simulink library "powerlib2"  (Simulink 6.0)
settings: Solver=ode45  SolverMode=SingleTasking  StartTime=0.0  StopTime=10.0  RelTol=1e-3
undefined symbols (not defined in the file or in its folder): com, ctrl1, Da, DiscIntNeverNeededParam, dtha, etat, FA, gcbh, Ha, Ka, Lm, Ls, powericonV2, q0, Rm, Rs, sel, st_a, st_b, st_c, sta, stb, stc, T1, T2, T3, T4
libraries: powerlib2 x55, simulink_extras x5, powerlib_extras x4, powerlib_modelsV2 x4, simulink x1
(part 6 of 6)

== system powerlib2/Machines/STG/4 mass shaft/2 masses/Mass2 ==
  Ts_k+1 : Inport  Port=1  LatchInput=off
  Tt_k : Inport  Port=2  LatchInput=off
  deltat_k-1 : Inport  Port=3  LatchInput=off
  Gain10 : Gain  Gain=D  SaturateOnIntegerOverflow=on
  Gain11 : Gain  Gain=K  SaturateOnIntegerOverflow=on
  Gain9 : Gain  Gain=1/(2*H)  SaturateOnIntegerOverflow=on
  Integrator6 : Integrator
  Integrator7 : Integrator  InitialCondition=dth0
  Sum11 : Sum  Orientation=left  Inputs=|+-  SaturateOnIntegerOverflow=on  InputSameDT=on
  Sum9 : Sum  Inputs=+|+|-|-  SaturateOnIntegerOverflow=on  InputSameDT=on
  pu2radpersec : Gain  Gain=120*pi  SaturateOnIntegerOverflow=on
  deltat_k : Outport  InitialOutput=0
  Ts_k : Outport  Port=2  InitialOutput=0
  dw : Outport  Port=3  InitialOutput=0
  wires:
  deltat_k-1/1 -> Sum11/2
  Sum11/1 -> Gain11/1
  Integrator7/1 -> deltat_k/1, Sum11/1
  pu2radpersec/1 -> Integrator7/1
  Integrator6/1 -> pu2radpersec/1, Gain10/1, dw/1
  Tt_k/1 -> Sum9/2
  Sum9/1 -> Gain9/1
  Gain10/1 -> Sum9/4
  Gain11/1 -> Ts_k/1, Sum9/3
  Ts_k+1/1 -> Sum9/1
  Gain9/1 -> Integrator6/1

== system powerlib2/Machines/STG/4 mass shaft/2 masses/Mass3 ==
  Ts_k+1 : Inport  Port=1  LatchInput=off
  Tt_k : Inport  Port=2  LatchInput=off
  deltat_k-1 : Inport  Port=3  LatchInput=off
  Gain10 : Gain  Gain=D  SaturateOnIntegerOverflow=on
  Gain11 : Gain  Gain=K  SaturateOnIntegerOverflow=on
  Gain9 : Gain  Gain=1/(2*H)  SaturateOnIntegerOverflow=on
  Integrator6 : Integrator
  Integrator7 : Integrator  InitialCondition=dth0
  Sum11 : Sum  Orientation=left  Inputs=|+-  SaturateOnIntegerOverflow=on  InputSameDT=on
  Sum9 : Sum  Inputs=+|+|-|-  SaturateOnIntegerOverflow=on  InputSameDT=on
  pu2radpersec : Gain  Gain=120*pi  SaturateOnIntegerOverflow=on
  deltat_k : Outport  InitialOutput=0
  Ts_k : Outport  Port=2  InitialOutput=0
  dw : Outport  Port=3  InitialOutput=0
  wires:
  Ts_k+1/1 -> Sum9/1
  Gain11/1 -> Sum9/3, Ts_k/1
  Gain10/1 -> Sum9/4
  Sum9/1 -> Gain9/1
  Gain9/1 -> Integrator6/1
  Tt_k/1 -> Sum9/2
  Integrator6/1 -> pu2radpersec/1, Gain10/1, dw/1
  pu2radpersec/1 -> Integrator7/1
  Integrator7/1 -> Sum11/1, deltat_k/1
  Sum11/1 -> Gain11/1
  deltat_k-1/1 -> Sum11/2

== system powerlib2/Machines/STG/4 mass shaft/3 masses/Mass2 ==
  Ts_k+1 : Inport  Port=1  LatchInput=off
  Tt_k : Inport  Port=2  LatchInput=off
  deltat_k-1 : Inport  Port=3  LatchInput=off
  Gain10 : Gain  Gain=D  SaturateOnIntegerOverflow=on
  Gain11 : Gain  Gain=K  SaturateOnIntegerOverflow=on
  Gain9 : Gain  Gain=1/(2*H)  SaturateOnIntegerOverflow=on
  Integrator6 : Integrator
  Integrator7 : Integrator  InitialCondition=dth0
  Sum11 : Sum  Orientation=left  Inputs=|+-  SaturateOnIntegerOverflow=on  InputSameDT=on
  Sum9 : Sum  Inputs=+|+|-|-  SaturateOnIntegerOverflow=on  InputSameDT=on
  pu2radpersec : Gain  Gain=120*pi  SaturateOnIntegerOverflow=on
  deltat_k : Outport  InitialOutput=0
  Ts_k : Outport  Port=2  InitialOutput=0
  dw : Outport  Port=3  InitialOutput=0
  wires:
  deltat_k-1/1 -> Sum11/2
  Sum11/1 -> Gain11/1
  Integrator7/1 -> deltat_k/1, Sum11/1
  pu2radpersec/1 -> Integrator7/1
  Integrator6/1 -> pu2radpersec/1, Gain10/1, dw/1
  Tt_k/1 -> Sum9/2
  Sum9/1 -> Gain9/1
  Gain10/1 -> Sum9/4
  Gain11/1 -> Ts_k/1, Sum9/3
  Ts_k+1/1 -> Sum9/1
  Gain9/1 -> Integrator6/1

== system powerlib2/Machines/STG/4 mass shaft/3 masses/Mass3 ==
  Ts_k+1 : Inport  Port=1  LatchInput=off
  Tt_k : Inport  Port=2  LatchInput=off
  deltat_k-1 : Inport  Port=3  LatchInput=off
  Gain10 : Gain  Gain=D  SaturateOnIntegerOverflow=on
  Gain11 : Gain  Gain=K  SaturateOnIntegerOverflow=on
  Gain9 : Gain  Gain=1/(2*H)  SaturateOnIntegerOverflow=on
  Integrator6 : Integrator
  Integrator7 : Integrator  InitialCondition=dth0
  Sum11 : Sum  Orientation=left  Inputs=|+-  SaturateOnIntegerOverflow=on  InputSameDT=on
  Sum9 : Sum  Inputs=+|+|-|-  SaturateOnIntegerOverflow=on  InputSameDT=on
  pu2radpersec : Gain  Gain=120*pi  SaturateOnIntegerOverflow=on
  deltat_k : Outport  InitialOutput=0
  Ts_k : Outport  Port=2  InitialOutput=0
  dw : Outport  Port=3  InitialOutput=0
  wires:
  Ts_k+1/1 -> Sum9/1
  Gain11/1 -> Sum9/3, Ts_k/1
  Gain10/1 -> Sum9/4
  Sum9/1 -> Gain9/1
  Gain9/1 -> Integrator6/1
  Tt_k/1 -> Sum9/2
  Integrator6/1 -> pu2radpersec/1, Gain10/1, dw/1
  pu2radpersec/1 -> Integrator7/1
  Integrator7/1 -> Sum11/1, deltat_k/1
  Sum11/1 -> Gain11/1
  deltat_k-1/1 -> Sum11/2

== system powerlib2/Machines/STG/4 mass shaft/3 masses/Mass4 ==
  Ts_k+1 : Inport  Port=1  LatchInput=off
  Tt_k : Inport  Port=2  LatchInput=off
  deltat_k-1 : Inport  Port=3  LatchInput=off
  Gain10 : Gain  Gain=D  SaturateOnIntegerOverflow=on
  Gain11 : Gain  Gain=K  SaturateOnIntegerOverflow=on
  Gain9 : Gain  Gain=1/(2*H)  SaturateOnIntegerOverflow=on
  Integrator6 : Integrator
  Integrator7 : Integrator  InitialCondition=dth0
  Sum11 : Sum  Orientation=left  Inputs=|+-  SaturateOnIntegerOverflow=on  InputSameDT=on
  Sum9 : Sum  Inputs=+|+|-|-  SaturateOnIntegerOverflow=on  InputSameDT=on
  pu2radpersec : Gain  Gain=120*pi  SaturateOnIntegerOverflow=on
  deltat_k : Outport  InitialOutput=0
  Ts_k : Outport  Port=2  InitialOutput=0
  dw : Outport  Port=3  InitialOutput=0
  wires:
  deltat_k-1/1 -> Sum11/2
  Sum11/1 -> Gain11/1
  Integrator7/1 -> deltat_k/1, Sum11/1
  pu2radpersec/1 -> Integrator7/1
  Integrator6/1 -> pu2radpersec/1, Gain10/1, dw/1
  Tt_k/1 -> Sum9/2
  Gain9/1 -> Integrator6/1
  Sum9/1 -> Gain9/1
  Gain10/1 -> Sum9/4
  Gain11/1 -> Ts_k/1, Sum9/3
  Ts_k+1/1 -> Sum9/1

== system powerlib2/Machines/STG/4 mass shaft/4 masses/Mass2 ==
  Ts_k+1 : Inport  Port=1  LatchInput=off
  Tt_k : Inport  Port=2  LatchInput=off
  deltat_k-1 : Inport  Port=3  LatchInput=off
  Gain10 : Gain  Gain=D  SaturateOnIntegerOverflow=on
  Gain11 : Gain  Gain=K  SaturateOnIntegerOverflow=on
  Gain9 : Gain  Gain=1/(2*H)  SaturateOnIntegerOverflow=on
  Integrator6 : Integrator
  Integrator7 : Integrator  InitialCondition=dth0
  Sum11 : Sum  Orientation=left  Inputs=|+-  SaturateOnIntegerOverflow=on  InputSameDT=on
  Sum9 : Sum  Inputs=+|+|-|-  SaturateOnIntegerOverflow=on  InputSameDT=on
  pu2radpersec : Gain  Gain=120*pi  SaturateOnIntegerOverflow=on
  deltat_k : Outport  InitialOutput=0
  Ts_k : Outport  Port=2  InitialOutput=0
  dw : Outport  Port=3  InitialOutput=0
  wires:
  Gain9/1 -> Integrator6/1
  Ts_k+1/1 -> Sum9/1
  Gain11/1 -> Sum9/3, Ts_k/1
  Gain10/1 -> Sum9/4
  Sum9/1 -> Gain9/1
  Tt_k/1 -> Sum9/2
  Integrator6/1 -> pu2radpersec/1, Gain10/1, dw/1
  pu2radpersec/1 -> Integrator7/1
  Integrator7/1 -> Sum11/1, deltat_k/1
  Sum11/1 -> Gain11/1
  deltat_k-1/1 -> Sum11/2

== system powerlib2/Machines/STG/4 mass shaft/4 masses/Mass3 ==
  Ts_k+1 : Inport  Port=1  LatchInput=off
  Tt_k : Inport  Port=2  LatchInput=off
  deltat_k-1 : Inport  Port=3  LatchInput=off
  Gain10 : Gain  Gain=D  SaturateOnIntegerOverflow=on
  Gain11 : Gain  Gain=K  SaturateOnIntegerOverflow=on
  Gain9 : Gain  Gain=1/(2*H)  SaturateOnIntegerOverflow=on
  Integrator6 : Integrator
  Integrator7 : Integrator  InitialCondition=dth0
  Sum11 : Sum  Orientation=left  Inputs=|+-  SaturateOnIntegerOverflow=on  InputSameDT=on
  Sum9 : Sum  Inputs=+|+|-|-  SaturateOnIntegerOverflow=on  InputSameDT=on
  pu2radpersec : Gain  Gain=120*pi  SaturateOnIntegerOverflow=on
  deltat_k : Outport  InitialOutput=0
  Ts_k : Outport  Port=2  InitialOutput=0
  dw : Outport  Port=3  InitialOutput=0
  wires:
  deltat_k-1/1 -> Sum11/2
  Sum11/1 -> Gain11/1
  Integrator7/1 -> deltat_k/1, Sum11/1
  pu2radpersec/1 -> Integrator7/1
  Integrator6/1 -> pu2radpersec/1, Gain10/1, dw/1
  Tt_k/1 -> Sum9/2
  Gain9/1 -> Integrator6/1
  Sum9/1 -> Gain9/1
  Gain10/1 -> Sum9/4
  Gain11/1 -> Ts_k/1, Sum9/3
  Ts_k+1/1 -> Sum9/1

== system powerlib2/Machines/STG/4 mass shaft/4 masses/Mass4 ==
  Ts_k+1 : Inport  Port=1  LatchInput=off
  Tt_k : Inport  Port=2  LatchInput=off
  deltat_k-1 : Inport  Port=3  LatchInput=off
  Gain10 : Gain  Gain=D  SaturateOnIntegerOverflow=on
  Gain11 : Gain  Gain=K  SaturateOnIntegerOverflow=on
  Gain9 : Gain  Gain=1/(2*H)  SaturateOnIntegerOverflow=on
  Integrator6 : Integrator
  Integrator7 : Integrator  InitialCondition=dth0
  Sum11 : Sum  Orientation=left  Inputs=|+-  SaturateOnIntegerOverflow=on  InputSameDT=on
  Sum9 : Sum  Inputs=+|+|-|-  SaturateOnIntegerOverflow=on  InputSameDT=on
  pu2radpersec : Gain  Gain=120*pi  SaturateOnIntegerOverflow=on
  deltat_k : Outport  InitialOutput=0
  Ts_k : Outport  Port=2  InitialOutput=0
  dw : Outport  Port=3  InitialOutput=0
  wires:
  Ts_k+1/1 -> Sum9/1
  Gain11/1 -> Sum9/3, Ts_k/1
  Gain10/1 -> Sum9/4
  Sum9/1 -> Gain9/1
  Gain9/1 -> Integrator6/1
  Tt_k/1 -> Sum9/2
  Integrator6/1 -> pu2radpersec/1, Gain10/1, dw/1
  pu2radpersec/1 -> Integrator7/1
  Integrator7/1 -> Sum11/1, deltat_k/1
  Sum11/1 -> Gain11/1
  deltat_k-1/1 -> Sum11/2

== system powerlib2/Machines/STG/4 mass shaft/4 masses/Mass5 ==
  Ts_k+1 : Inport  Port=1  LatchInput=off
  Tt_k : Inport  Port=2  LatchInput=off
  deltat_k-1 : Inport  Port=3  LatchInput=off
  Gain10 : Gain  Gain=D  SaturateOnIntegerOverflow=on
  Gain11 : Gain  Gain=K  SaturateOnIntegerOverflow=on
  Gain9 : Gain  Gain=1/(2*H)  SaturateOnIntegerOverflow=on
  Integrator6 : Integrator
  Integrator7 : Integrator  InitialCondition=dth0
  Sum11 : Sum  Orientation=left  Inputs=|+-  SaturateOnIntegerOverflow=on  InputSameDT=on
  Sum9 : Sum  Inputs=+|+|-|-  SaturateOnIntegerOverflow=on  InputSameDT=on
  pu2radpersec : Gain  Gain=120*pi  SaturateOnIntegerOverflow=on
  deltat_k : Outport  InitialOutput=0
  Ts_k : Outport  Port=2  InitialOutput=0
  dw : Outport  Port=3  InitialOutput=0
  wires:
  deltat_k-1/1 -> Sum11/2
  Sum11/1 -> Gain11/1
  Integrator7/1 -> deltat_k/1, Sum11/1
  pu2radpersec/1 -> Integrator7/1
  Integrator6/1 -> pu2radpersec/1, Gain10/1, dw/1
  Tt_k/1 -> Sum9/2
  Gain9/1 -> Integrator6/1
  Sum9/1 -> Gain9/1
  Gain10/1 -> Sum9/4
  Gain11/1 -> Ts_k/1, Sum9/3
  Ts_k+1/1 -> Sum9/1

== system powerlib2/Machines/STG/steam turbine/Stage1/Stage4 ==
  In1 : Inport  Port=1  LatchInput=off
  Enable : EnablePort
  Transfer Fcn (with initial outputs)3 : simulink_extras/Additional Linear/Transfer Fcn (with initial outputs)  N=[1]  D="[T4  1]"  Y0=f0  U0=f0
  Out1 : Outport  OutputWhenDisabled=reset  InitialOutput=0
  wires:
  In1/1 -> Transfer Fcn (with initial outputs)3/1
  Transfer Fcn (with initial outputs)3/1 -> Out1/1

== system powerlib2/Machines/STG/steam turbine/Stage2/Stage3 ==
  In1 : Inport  Port=1  LatchInput=off
  Enable : EnablePort
  Transfer Fcn (with initial outputs)3 : simulink_extras/Additional Linear/Transfer Fcn (with initial outputs)  N=[1]  D="[T3  1]"  Y0=f0  U0=f0
  Out1 : Outport  OutputWhenDisabled=reset  InitialOutput=0
  wires:
  Transfer Fcn (with initial outputs)3/1 -> Out1/1
  In1/1 -> Transfer Fcn (with initial outputs)3/1

== system powerlib2/Machines/STG/steam turbine/Stage3 /Stage2 ==
  In1 : Inport  Port=1  LatchInput=off
  Enable : EnablePort
  Transfer Fcn (with initial outputs)3 : simulink_extras/Additional Linear/Transfer Fcn (with initial outputs)  N=[1]  D="[T2  1]"  Y0=f0  U0=f0
  Out1 : Outport  OutputWhenDisabled=reset  InitialOutput=0
  wires:
  In1/1 -> Transfer Fcn (with initial outputs)3/1
  Transfer Fcn (with initial outputs)3/1 -> Out1/1

== system powerlib2/Machines/STG/steam turbine/Stage4/Stage1 ==
  In1 : Inport  Port=1  LatchInput=off
  Enable : EnablePort
  Transfer Fcn (with initial outputs)3 : simulink_extras/Additional Linear/Transfer Fcn (with initial outputs)  N=[1]  D="[T1  1]"  Y0=f0  U0=f0
  Out1 : Outport  OutputWhenDisabled=reset  InitialOutput=0
  wires:
  Transfer Fcn (with initial outputs)3/1 -> Out1/1
  In1/1 -> Transfer Fcn (with initial outputs)3/1
